simulink model "wpt_circuit"  (R2022b)
settings: Solver=VariableStepAuto  StartTime=0.0  StopTime=1  RelTol=1e-3
undefined symbols (not defined in the file): Ion, Lithium
libraries: spsMosfetLib x8, spsCurrentMeasurementLib x5, spsVoltageMeasurementLib x5, spsSeriesRLCBranchLib x4, eePowerMeasurement x2, spsUniversalBridgeLib x2, spsACVoltageSourceLib x1, spsBatteryLib x1, spsDiodeLib x1, spsMutualInductanceLib x1, spspowerguiLib x1
settings Model: Creator=AKHIL  LastModifiedBy=AKHIL
settings SolverCC: ZeroCrossAlgorithm=Adaptive
settings DebuggingCC: IgnoredZcDiagnostic=none

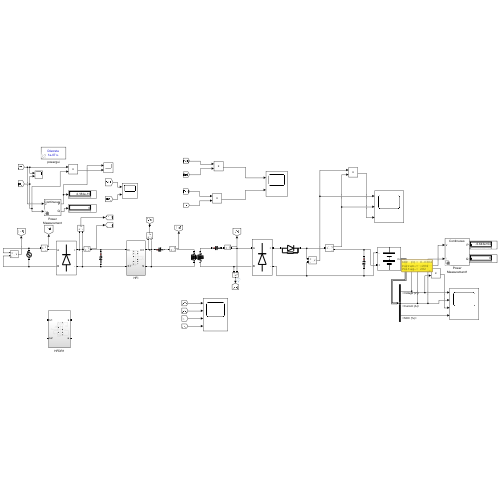
[thumbnail: Simulink's stored preview of the top-level diagram]
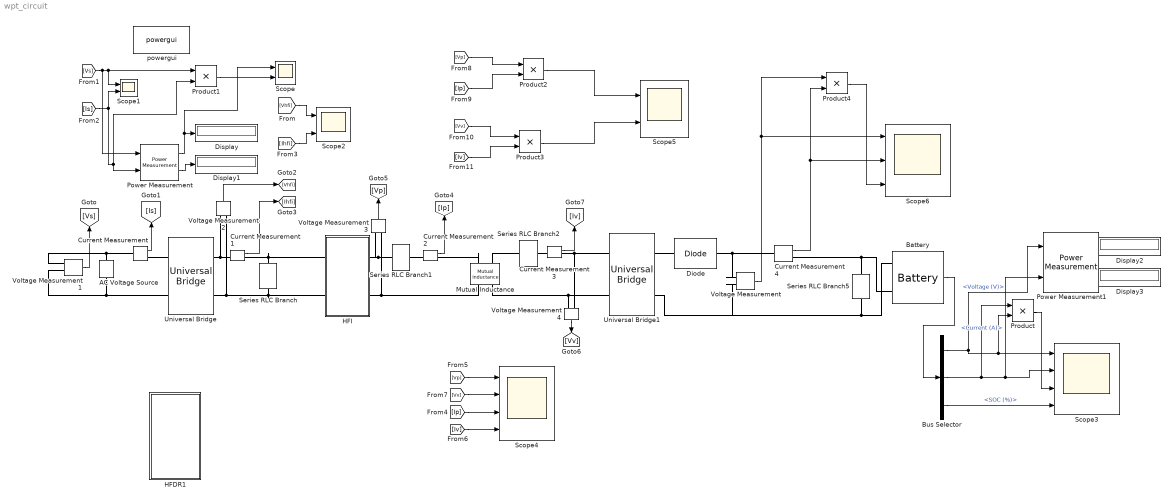
== system wpt_circuit ==
  AC Voltage Source : spsACVoltageSourceLib/AC Voltage Source  Amplitude=325  Phase=0  Frequency=50  SampleTime=0  Measurements=None  BusType=swing  Pref=10e3  Qref=0  Qmin=-inf  Qmax=+inf
  Battery : spsBatteryLib/Battery  BatType=Lithium-Ion  ShowTempParam=off  ThermalPreset=no  ShowAgeParam=off  NomV=320  NomQ=94.5  SOC=0  Batt_Tr=30  PresetModel=on  MaxQ=94.5  MinV=240  FullV=372.4759  Dis_rate=41.087  R=0.033862  Normal_OP=85.4609  expZone="[345.7235      4.642826]"  current=[6.5 13 32.5]  Units=Time  Tci=20  NomT=20  T2=-30  MaxQ2=4.8  FullV2=7.1  Normal_OP2=5.655  expZone2="[6.58           1]"  Rca=0.6  ti=2000  Dp=0  Neq0=0  Tsim=1e6  Ta1=25  Qeol=5.4*0.9  Reol=0.013333*1.2  Char_age=[2.3478, 3]  Dis_age=[2.3478, 10]  N1=1500  N2=10500  N3=1000  N4=1400  Ta2=45  N5=950
  Bus Selector : BusSelector  OutputSignals=Voltage (V),Current (A),SOC (%)
  Current Measurement{,1..4} (5 alike) : spsCurrentMeasurementLib/Current Measurement  PhasorSimulation=off  OutputType=Complex  PSBequivalent=0
  Diode : spsDiodeLib/Diode  Ron=0.001  Lon=0  Vf=0.8  IC=0  UseSnubber=0  Rs=500  Cs=250e-9  Measurements=off
  Display{,1..3} (4 alike) : Display
  HFDR1 : Subsystem
  HFI : Subsystem
  Mutual Inductance : spsMutualInductanceLib/Mutual Inductance  LConnTagsString=a|b  RConnTagsString=A|B  TypeOfMutual=Two or three windings with equal mutual terms  NumberOfWindings=3  SelfImpedance1=[1e-3 4.27e-6]  SelfImpedance2=[ 1e-3 4.27e-6]  ThreeWindings=off  SelfImpedance3=[ 1.1 1.1e-03]  MutualImpedance=[0 2e-6]  InductanceMatrix="[1.0 0.9  0.9 ;  0.9 1.0  0.9;  0.9 0.9 1.0 ] * 1e-3"  ResistanceMatrix="[1.0 0.9  0.9 ;  0.9 1.0  0.9;  0.9 0.9 1.0 ]"  Measurements=Winding voltages and currents
      settings: LibrarySourceBlock=sps_lib/Passives/Mutual Inductance
  Power Measurement : eePowerMeasurement/Power Measurement  LabelModeActiveChoice=Continuous  F=50  K=[0 1 2 3]  Ts=0
  Power Measurement1 : eePowerMeasurement/Power Measurement  LabelModeActiveChoice=Continuous  F=50  K=[0 1 2 3]  Ts=0
  Product{,1..4} (5 alike) : Product
  Scope{,1..2,5} (4 alike) : Scope  NumInputPorts=2
  Scope3 : Scope  NumInputPorts=4
  Scope4 : Scope  NumInputPorts=4
  Scope6 : Scope  NumInputPorts=3
  Series RLC Branch : spsSeriesRLCBranchLib/Series RLC Branch  LConnTagsString=__new0  RConnTagsString=__new0  BranchType=C  Resistance=10  Inductance=1e-3  SetiL0=off  InitialCurrent=0  Capacitance=0.22  Setx0=off  InitialVoltage=0  Measurements=None
  Series RLC Branch1 : spsSeriesRLCBranchLib/Series RLC Branch  LConnTagsString=__new0  RConnTagsString=__new0  BranchType=C  Resistance=1  Inductance=1e-3  SetiL0=off  InitialCurrent=0  Capacitance=0.8e-6  Setx0=off  InitialVoltage=0  Measurements=None
  Series RLC Branch2 : spsSeriesRLCBranchLib/Series RLC Branch  LConnTagsString=__new0  RConnTagsString=__new0  BranchType=C  Resistance=1  Inductance=1e-3  SetiL0=off  InitialCurrent=0  Capacitance=0.8e-6  Setx0=off  InitialVoltage=0  Measurements=None
  Series RLC Branch5 : spsSeriesRLCBranchLib/Series RLC Branch  LConnTagsString=__new0  RConnTagsString=__new0  BranchType=C  Resistance=10  Inductance=0.8e-6  SetiL0=off  InitialCurrent=0  Capacitance=1e-3  Setx0=off  InitialVoltage=0  Measurements=None
  Universal Bridge : spsUniversalBridgeLib/Universal Bridge  Arms=2  SnubberResistance=1e5  SnubberCapacitance=inf  Device=Diodes  Ron=1e-3  Lon=0  ForwardVoltages="[  0  0  ]"  ForwardVoltage=0  GTOparameters=[ 10e-6 , 20e-6 ]  IGBTparameters=[ 1e-6 , 2e-6 ]  Measurements=None  Measurements_2=None  converterType=Rectifier
  Universal Bridge1 : spsUniversalBridgeLib/Universal Bridge  Arms=2  SnubberResistance=1e5  SnubberCapacitance=inf  Device=Diodes  Ron=1e-3  Lon=0  ForwardVoltages="[  0  0  ]"  ForwardVoltage=0  GTOparameters=[ 10e-6 , 20e-6 ]  IGBTparameters=[ 1e-6 , 2e-6 ]  Measurements=None  Measurements_2=None  converterType=Rectifier
  Voltage Measurement{,1..4} (5 alike) : spsVoltageMeasurementLib/Voltage Measurement  PhasorSimulation=off  OutputType=Complex  PSBequivalent=0
  powergui : spspowerguiLib/powergui  Priority=1  SimulationMode=Discrete  SampleTime=1e-7  frequency=60  Iterations=50  frequencyindice=0  Pbase=100e6  ErrMax=1e-4  UnitsV=kV  UnitsW=MW  buscounter=0  FunctionMessages=off  echomessages=off  EnableUseOfTLC=off  CurrentSourceSwitches=off  DisableSnubberDevices=off  DisableRonSwitches=off  DisableVfSwitches=off  DisplayEquations=off  AutomaticDiscreteSolvers=off  SolverType=Tustin/Backward Euler (TBE)  Interpol=off  ExternalGateDelay=off  methode=off  Ts=100  x0status=blocks  SPID=on  SwTol=0  HookPort=off  NonlinearTolerance=1e-4  nMaxIteration=100  ContinueOnMaxIteration=off  RestoreLinks=warning  ResistiveCurrentMeasurement=off  Frange=[0:2:500]  Ylog=off  Xlog=on  ShowGrid=off  save=off  variable=ZData  structure=0  ZoomFFT=off  StartTime=0.0  cycles=1  DisplayStyle=1  fundamental=60  FreqAxis=off  MaxFrequency=1000  frequencyindicesteady=1  RmsSteady=1  display=off
  wires:
  Voltage Measurement1/1 -> [Vs]
  Current Measurement/1 -> [Is]
  [Is] -> Scope1/2, Product1/2, Power Measurement/2
  Current Measurement1/1 -> [Ihfi]
  [Vhfi] -> Scope2/1
  [Ihfi] -> Scope2/2
  Current Measurement2/1 -> [Ip]
  Voltage Measurement3/1 -> [Vp]
  [Ip] -> Scope4/3
  Voltage Measurement4/1 -> [Vv]
  Current Measurement3/1 -> [Iv]
  [Vv] -> Scope4/2
  [Iv] -> Scope4/4
  Battery/1 -> Bus Selector/1
  [Vp] -> Scope4/1
  Bus Selector/1 -> Power Measurement1/1, Scope3/1, Product/2  "<Voltage (V)>"
  Bus Selector/2 -> Product/1, Power Measurement1/2, Scope3/2  "<Current (A)>"
  Voltage Measurement2/1 -> [Vhfi]
  Product/1 -> Scope3/3
  Bus Selector/3 -> Scope3/4  "<SOC (%)>"
  [Vs] -> Product1/1, Scope1/1, Power Measurement/1
  Power Measurement/1 -> Scope/1, Display/1
  Power Measurement/2 -> Display1/1
  Power Measurement1/1 -> Display2/1
  Power Measurement1/2 -> Display3/1
  Product1/1 -> Scope/2
  [Vp] -> Product2/1
  [Ip] -> Product2/2
  [Vv] -> Product3/1
  [Iv] -> Product3/2
  Product2/1 -> Scope5/1
  Product3/1 -> Scope5/2
  Product4/1 -> Scope6/3
  Current Measurement4/1 -> Product4/2, Scope6/2
  Voltage Measurement/1 -> Scope6/1, Product4/1
  connections:
  Current Measurement/LConn1 -- Voltage Measurement1/LConn1 -- AC Voltage Source/RConn1
  HFI/LConn2 -- Series RLC Branch/RConn1 -- Voltage Measurement2/LConn2 -- Universal Bridge/RConn2
  HFI/RConn2 -- Mutual Inductance/RConn1 -- Voltage Measurement3/LConn2
  Voltage Measurement4/LConn1 -- Universal Bridge1/LConn1 -- Current Measurement3/RConn1
  Mutual Inductance/RConn2 -- Voltage Measurement4/LConn2 -- Universal Bridge1/LConn2
  Series RLC Branch1/LConn1 -- Voltage Measurement3/LConn1 -- HFI/RConn1
  Universal Bridge/LConn1 -- Current Measurement/RConn1
  Voltage Measurement2/LConn1 -- Universal Bridge/RConn1 -- Current Measurement1/LConn1
  Current Measurement2/LConn1 -- Series RLC Branch1/RConn1
  Series RLC Branch2/RConn1 -- Current Measurement3/LConn1
  HFI/LConn1 -- Series RLC Branch/LConn1 -- Current Measurement1/RConn1
  Mutual Inductance/LConn2 -- Series RLC Branch2/LConn1
  Mutual Inductance/LConn1 -- Current Measurement2/RConn1
  Series RLC Branch5/RConn1 -- Voltage Measurement/LConn2 -- Universal Bridge1/RConn2 -- Battery/LConn2
  AC Voltage Source/LConn1 -- Voltage Measurement1/LConn2 -- Universal Bridge/LConn2
  Series RLC Branch5/LConn1 -- Current Measurement4/RConn1 -- Battery/LConn1
  Universal Bridge1/RConn1 -- Diode/LConn1
  Current Measurement4/LConn1 -- Voltage Measurement/LConn1 -- Diode/RConn1

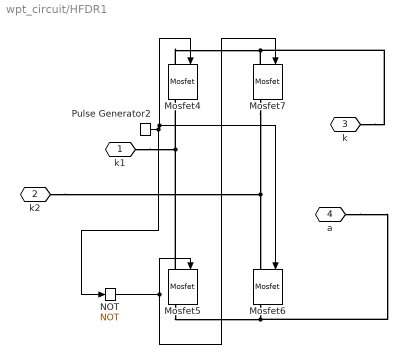
== system wpt_circuit/HFDR1 ==
  Mosfet{4..7} (4 alike) : spsMosfetLib/Mosfet  Ron=0.1  Lon=0  Rd=0.01  Vfd=0  IC=0  Rs=1e5  Cs=inf  Measurements=on
  NOT : Logic  Operator=NOT  IconShape=distinctive  AllPortsSameDT=off  OutDataTypeStr=boolean
  Pulse Generator2 : DiscretePulseGenerator  PulseType=Time based  Period=1/85000  PulseWidth=50
  k1 : PMIOPort  Side=Left
  k2 : PMIOPort  Port=2  Side=Left
  k : PMIOPort  Port=3  Side=Right
  a : PMIOPort  Port=4  Side=Right
  wires:
  Pulse Generator2/1 -> NOT/1, Mosfet6/1, Mosfet4/1
  NOT/1 -> Mosfet5/1, Mosfet7/1
  connections:
  Mosfet4/LConn1 -- k/RConn1 -- Mosfet7/LConn1
  Mosfet5/RConn1 -- a/RConn1 -- Mosfet6/RConn1
  Mosfet5/LConn1 -- k1/RConn1 -- Mosfet4/RConn1
  Mosfet7/RConn1 -- k2/RConn1 -- Mosfet6/LConn1

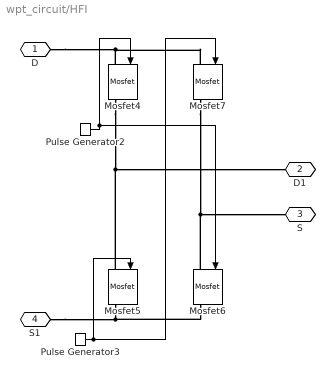
== system wpt_circuit/HFI ==
  Mosfet{4..7} (4 alike) : spsMosfetLib/Mosfet  Ron=0.1  Lon=0  Rd=0.01  Vfd=0  IC=0  Rs=1e5  Cs=inf  Measurements=on
  Pulse Generator2 : DiscretePulseGenerator  PulseType=Time based  Period=1/85000  PulseWidth=50
  Pulse Generator3 : DiscretePulseGenerator  PulseType=Time based  Period=1/85000  PulseWidth=50  PhaseDelay=1/(2*85000)
  D : PMIOPort  Side=Left
  D1 : PMIOPort  Port=2  Side=Right
  S : PMIOPort  Port=3  Side=Right
  S1 : PMIOPort  Port=4  Side=Left
  wires:
  Pulse Generator3/1 -> Mosfet7/1, Mosfet5/1
  Pulse Generator2/1 -> Mosfet6/1, Mosfet4/1
  connections:
  Mosfet6/LConn1 -- S/RConn1 -- Mosfet7/RConn1
  Mosfet4/RConn1 -- D1/RConn1 -- Mosfet5/LConn1
  Mosfet6/RConn1 -- S1/RConn1 -- Mosfet5/RConn1
  Mosfet7/LConn1 -- D/RConn1 -- Mosfet4/LConn1
